simulink model "Sim_Helikopter_FB_VS"  (R2020b)
settings: Solver=ode113  StartTime=0.0  StopTime=50  RelTol=1e-2  EnableMultiTasking=on
PostLoadFcn:
  | , if any(exist('dsrtsu_mdlpostloadfcn', 'file') == [2, 3, 6]), try dsrtsu_mdlpostloadfcn('Execute', bdroot); catch fprintf('Error in PostLoadFcn (dsrtsu_mdlpostloadfcn) for model "%s":\n %s\n', bdroot, lasterr); end, end,
values from neighbouring files (symbols this model uses):
  Ta = 1e-3    (= 0.001)    [Initialisierung_bitte_vervollstaendigen.m]
undefined symbols (not defined in the file or in its folder): fbvsPar, initCond, sysPar
settings Model: DSRTSU_INTERNAL_RTI_VER=480  DSRTSU_INTERNAL_RTI_TYPE=rti1202  DSRTSU_INTERNAL_RTIFPGA=70  ExtModeArmWhenConnect=off  Creator=tk  LastModifiedBy=simon
settings DataIOCC: LimitDataPoints=on  SaveFormat=Array  SignalLoggingSaveFormat=ModelDataLogs  ReturnWorkspaceOutputs=off  SignalLoggingName=sigsOut
settings OptimizationCC: ConditionallyExecuteInputs=off  OptimizeBlockIOStorage=off  BufferReuse=off  GlobalBufferReuse=off  ExpressionFolding=off  ExpressionDepthLimit=2147483647  LocalBlockOutputs=off  InitFltsAndDblsToZero=on  LifeSpan=inf  OptimizeDataStoreBuffers=off  BusAssignmentInplaceUpdate=off
settings DebuggingCC: SaveWithParameterizedLinksMsg=none  UnderspecifiedInitializationDetection=Classic  MergeDetectMultiDrivingBlocksExec=none  SignalResolutionControl=TryResolveAllWithWarning  MultiTaskDSMMsg=warning  MultiTaskCondExecSysMsg=none  FcnCallInpInsideContextMsg=warning  AllowSymbolicDim=off  StateNameClashWarn=warning  SFUnexpectedBacktrackingDiag=warning  SFNoUnconditionalDefaultTransitionDiag=warning  SFExecutionAtInitializationDiag=none  ArithmeticOperatorsInVariantConditions=warning
settings HardwareCC: ProdBitPerPointer=32  ProdBitPerSizeT=32  ProdBitPerPtrDiffT=32  ProdLargestAtomicFloat=None  ProdIntDivRoundTo=Undefined  ProdEndianess=Unspecified  ProdWordSize=32  ProdHWDeviceType=32-bit Generic  TargetBitPerLong=64  TargetBitPerPointer=64  TargetBitPerSizeT=64  TargetBitPerPtrDiffT=64  TargetLongLongMode=on  TargetIntDivRoundTo=Zero  TargetEndianess=LittleEndian  TargetWordSize=64  TargetHWDeviceType=MATLAB Host  ProdEqTarget=off
settings ModelReferenceCC: PropagateSignalLabelsOutOfModel=off
settings SFSimCC: SimUseLocalCustomCode=off  SimParseCustomCode=off  CustomCodeUndefinedFunction=UseInterfaceOnly
settings RTWCC: Description=S-function Target  SystemTargetFile=rtwsfcn.tlc  TemplateMakefile=rtwsfcn_default_tmf  RetainRTWFile=on  RTWUseLocalCustomCode=off  RTWCompilerOptimization=on
settings CodeAppCC: StateflowObjectComments=on
settings STFCustomTargetCC: ModelReferenceCompliant=off  CompOptLevelCompliant=on  ConcurrentExecutionCompliant=off  MATLABClassNameForMDSCustomization=Simulink.SoftwareTarget.TargetSpecificTriggerConfigurationBase  CPPClassGenCompliant=off  SystemTargetFile=rtwsfcn.tlc
settings ConfigComp: CovMetricSettings=dw  CovSaveCumulativeToWorkspaceVar=on  CovSaveSingleToWorkspaceVar=on  CovExternalEMLEnable=off

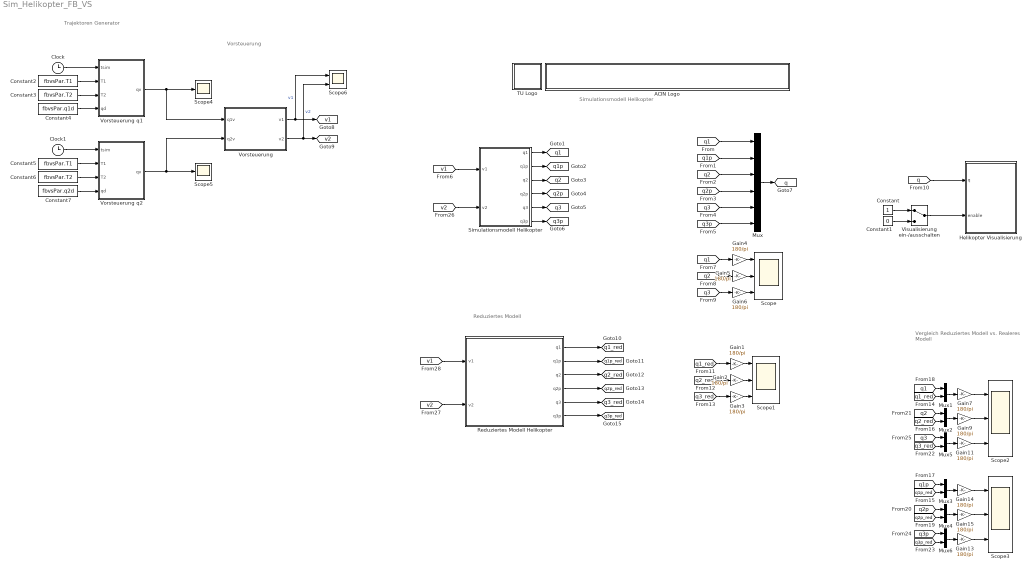
== system Sim_Helikopter_FB_VS ==
  note: Simulationsmodell Helikopter
  note: Reduziertes Modell
  note: Vergleich
      | Reduziertes Modell vs.
      | Realeres Modell
  note: Trajektoren
      | Generator
  note: Vorsteuerung
  ACIN Logo : Subsystem
      mask init:
      | s = get_param(gcb,'UserData');
      mask Display:
      | image(s.logo,[0 0 439 45]);
      | %axis image
  Clock : Clock
  Clock1 : Clock
  Constant : Constant
  Constant1 : Constant  Value=0
  Constant2 : Constant  Value=fbvsPar.T1
  Constant3 : Constant  Value=fbvsPar.T2
  Constant4 : Constant  Value=fbvsPar.q1d
  Constant5 : Constant  Value=fbvsPar.T1
  Constant6 : Constant  Value=fbvsPar.T2
  Constant7 : Constant  Value=fbvsPar.q2d
  Gain{1..7,9,11,13..15} (12 alike) : Gain  Gain=180/pi  SaturateOnIntegerOverflow=on  OutDataTypeStr=Inherit: Same as input  ParamDataTypeStr=Inherit: Same as input
  Helikopter Visualisierung : MATLAB Function  TreatAsAtomicUnit=on
  Mux : Mux  Inputs=6
  Mux{1..6} (6 alike) : Mux  Inputs=2
  Reduziertes Modell Helikopter : MATLAB Function  TreatAsAtomicUnit=on
  Scope{,1..3} (4 alike) : Scope  NumInputPorts=3
  Scope4 : Scope
  Scope5 : Scope
  Scope6 : Scope  NumInputPorts=2
  Simulationsmodell Helikopter : Subsystem
      settings: MinAlgLoopOccurrences=on
  TU Logo : Subsystem
      mask init:
      | s = get_param(gcb,'UserData');
      mask Display: image(s.logo,[0 0 45 45]);
  Visualisierung ein-/ausschalten : ManualSwitch
  Vorsteuerung : MATLAB Function  TreatAsAtomicUnit=on
  Vorsteuerung q1 : MATLAB Function  TreatAsAtomicUnit=on
  Vorsteuerung q2 : MATLAB Function  TreatAsAtomicUnit=on
  tag scope: q1=global, q1_red=global, q1p=global, q1p_red=global, q2=global, q2_red=global, q2p=global, q2p_red=global, q3=global, q3_red=global, q3p=global, q3p_red=global, q=global, v1=global, v2=global
  wires:
  Gain4/1 -> Scope/1
  Gain5/1 -> Scope/2
  Gain6/1 -> Scope/3
  Vorsteuerung/1(v1) -> Scope6/1, [v1]  "v1"
  Vorsteuerung/2(v2) -> Scope6/2, [v2]  "v2"
  Simulationsmodell Helikopter/1(q1) -> [q1]
  Simulationsmodell Helikopter/2(q1p) -> [q1p]
  Simulationsmodell Helikopter/3(q2) -> [q2]
  Simulationsmodell Helikopter/4(q2p) -> [q2p]
  Simulationsmodell Helikopter/5(q3) -> [q3]
  Simulationsmodell Helikopter/6(q3p) -> [q3p]
  Mux/1 -> [q]
  [q1] -> Mux/1
  [q1p] -> Mux/2
  [q2] -> Mux/3
  [q2p] -> Mux/4
  [q3] -> Mux/5
  [q3p] -> Mux/6
  [q1] -> Gain4/1
  [q2] -> Gain5/1
  [q3] -> Gain6/1
  Visualisierung ein-/ausschalten/1 -> Helikopter Visualisierung/2(enable)
  Constant/1 -> Visualisierung ein-/ausschalten/1
  [q] -> Helikopter Visualisierung/1(q)
  Constant1/1 -> Visualisierung ein-/ausschalten/2
  Reduziertes Modell Helikopter/1(q1) -> [q1_red]
  Reduziertes Modell Helikopter/2(q1p) -> [q1p_red]
  Reduziertes Modell Helikopter/3(q2) -> [q2_red]
  Reduziertes Modell Helikopter/4(q2p) -> [q2p_red]
  Reduziertes Modell Helikopter/5(q3) -> [q3_red]
  Reduziertes Modell Helikopter/6(q3p) -> [q3p_red]
  Gain1/1 -> Scope1/1
  [q1_red] -> Gain1/1
  Gain2/1 -> Scope1/2
  [q2_red] -> Gain2/1
  [q3_red] -> Gain3/1
  Gain3/1 -> Scope1/3
  Gain7/1 -> Scope2/1
  Mux1/1 -> Gain7/1
  [q1_red] -> Mux1/2
  [q1p_red] -> Mux3/2
  [q1p] -> Mux3/1
  [q1] -> Mux1/1
  [q2] -> Mux2/1
  [q2p] -> Mux4/1
  [q2_red] -> Mux2/2
  [q2p_red] -> Mux4/2
  [q3p_red] -> Mux6/2
  [q3p] -> Mux6/1
  [q3_red] -> Mux5/2
  [q3] -> Mux5/1
  Mux2/1 -> Gain9/1
  Mux5/1 -> Gain11/1
  Gain9/1 -> Scope2/2
  Gain11/1 -> Scope2/3
  Gain15/1 -> Scope3/2
  Gain14/1 -> Scope3/1
  Gain13/1 -> Scope3/3
  Mux3/1 -> Gain14/1
  Mux4/1 -> Gain15/1
  Mux6/1 -> Gain13/1
  [v1] -> Simulationsmodell Helikopter/1(v1)
  [v2] -> Simulationsmodell Helikopter/2(v2)
  [v1] -> Reduziertes Modell Helikopter/1(v1)
  [v2] -> Reduziertes Modell Helikopter/2(v2)
  Clock/1 -> Vorsteuerung q1/1(tsim)
  Constant2/1 -> Vorsteuerung q1/2(T1)
  Constant3/1 -> Vorsteuerung q1/3(T2)
  Constant4/1 -> Vorsteuerung q1/4(qd)
  Constant6/1 -> Vorsteuerung q2/3(T2)
  Clock1/1 -> Vorsteuerung q2/1(tsim)
  Constant5/1 -> Vorsteuerung q2/2(T1)
  Constant7/1 -> Vorsteuerung q2/4(qd)
  Vorsteuerung q1/1(qv) -> Vorsteuerung/1(q1v), Scope4/1
  Vorsteuerung q2/1(qv) -> Vorsteuerung/2(q2v), Scope5/1

== system Sim_Helikopter_FB_VS/ACIN Logo ==

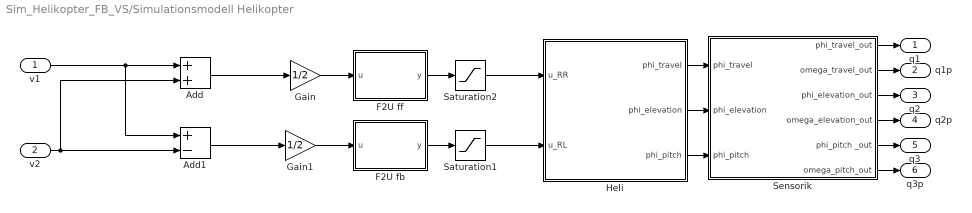
== system Sim_Helikopter_FB_VS/Simulationsmodell Helikopter ==
  v1 : Inport
  v2 : Inport  Port=2
  Add : Sum
  Add1 : Sum  Inputs=+-
  F2U fb : MATLAB Function  TreatAsAtomicUnit=on
  F2U ff : MATLAB Function  TreatAsAtomicUnit=on
  Gain : Gain  Gain=1/2
  Gain1 : Gain  Gain=1/2
  Heli : Subsystem
  Saturation1 : Saturate  UpperLimit=15  LowerLimit=-15
  Saturation2 : Saturate  UpperLimit=15  LowerLimit=-15
  Sensorik : Subsystem
  q1 : Outport  VectorParamsAs1DForOutWhenUnconnected=off
  q1p : Outport  Port=2  VectorParamsAs1DForOutWhenUnconnected=off
  q2 : Outport  Port=3  VectorParamsAs1DForOutWhenUnconnected=off
  q2p : Outport  Port=4  VectorParamsAs1DForOutWhenUnconnected=off
  q3 : Outport  Port=5  VectorParamsAs1DForOutWhenUnconnected=off
  q3p : Outport  Port=6  VectorParamsAs1DForOutWhenUnconnected=off
  wires:
  Saturation1/1 -> Heli/2(u_RL)
  Saturation2/1 -> Heli/1(u_RR)
  Heli/1(phi_travel) -> Sensorik/1(phi_travel)
  Heli/2(phi_elevation) -> Sensorik/2(phi_elevation)
  Heli/3(phi_pitch) -> Sensorik/3(phi_pitch)
  Sensorik/1(phi_travel_out) -> q1/1
  Sensorik/2(omega_travel_out) -> q1p/1
  Sensorik/3(phi_elevation_out) -> q2/1
  Sensorik/4(omega_elevation_out) -> q2p/1
  Sensorik/5(phi_pitch _out) -> q3/1
  Sensorik/6(omega_pitch_out) -> q3p/1
  v1/1 -> Add/1, Add1/1
  v2/1 -> Add/2, Add1/2
  Add/1 -> Gain/1
  Add1/1 -> Gain1/1
  Gain/1 -> F2U ff/1(u)
  Gain1/1 -> F2U fb/1(u)
  F2U ff/1(y) -> Saturation2/1
  F2U fb/1(y) -> Saturation1/1

== system Sim_Helikopter_FB_VS/TU Logo ==

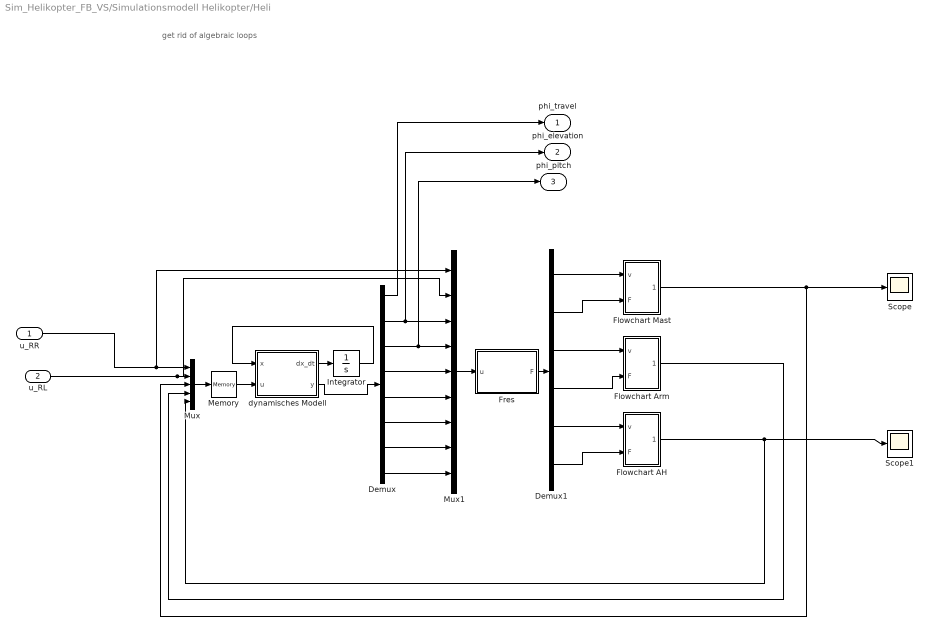
== system Sim_Helikopter_FB_VS/Simulationsmodell Helikopter/Heli ==
  note: get rid of algebraic loops
  u_RR : Inport
  u_RL : Inport  Port=2
  Demux : Demux  Outputs=8
      settings: DisplayOption=none
  Demux1 : Demux  Outputs=6
      settings: DisplayOption=none
  Flowchart AH : Subsystem
  Flowchart Arm : Subsystem
  Flowchart Mast : Subsystem
  Fres : MATLAB Function  TreatAsAtomicUnit=on
  Integrator : Integrator  InitialCondition=initCond
  Memory : Memory
  Mux : Mux  Inputs=5
  Mux1 : Mux  Inputs=9
  Scope : Scope
  Scope1 : Scope
  dynamisches Modell : MATLAB Function  TreatAsAtomicUnit=on
  phi_travel : Outport  VectorParamsAs1DForOutWhenUnconnected=off
  phi_elevation : Outport  Port=2  VectorParamsAs1DForOutWhenUnconnected=off
  phi_pitch : Outport  Port=3  VectorParamsAs1DForOutWhenUnconnected=off
  wires:
  Demux/1 -> phi_travel/1
  u_RR/1 -> Mux1/1, Mux/1
  u_RL/1 -> Mux1/2, Mux/2
  Demux1/6 -> Flowchart AH/2(F)
  Demux1/5 -> Flowchart AH/1(v)
  Demux1/4 -> Flowchart Arm/2(F)
  Demux1/3 -> Flowchart Arm/1(v)
  Demux1/2 -> Flowchart Mast/2(F)
  Demux1/1 -> Flowchart Mast/1(v)
  Fres/1(F) -> Demux1/1
  Mux1/1 -> Fres/1(u)
  Demux/2 -> Mux1/3, phi_elevation/1
  Demux/3 -> Mux1/4, phi_pitch/1
  Demux/4 -> Mux1/5
  Demux/5 -> Mux1/6
  Demux/6 -> Mux1/7
  Demux/7 -> Mux1/8
  Demux/8 -> Mux1/9
  dynamisches Modell/2(y) -> Demux/1
  Mux/1 -> Memory/1
  dynamisches Modell/1(dx_dt) -> Integrator/1
  Integrator/1 -> dynamisches Modell/1(x)
  Flowchart AH/1(Out1) -> Scope1/1, Mux/5
  Flowchart Arm/1(Out1) -> Mux/4
  Flowchart Mast/1(Out1) -> Mux/3, Scope/1
  Memory/1 -> dynamisches Modell/2(u)

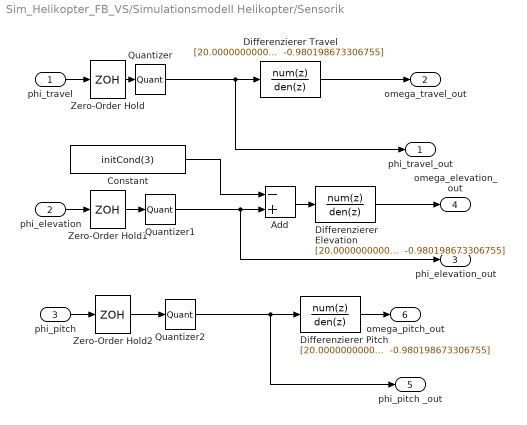
== system Sim_Helikopter_FB_VS/Simulationsmodell Helikopter/Sensorik ==
  phi_travel : Inport
  phi_elevation : Inport  Port=2
  phi_pitch : Inport  Port=3
  Add : Sum  Inputs=-+
  Constant : Constant  Value=initCond(3)
  Differenzierer Elevation : DiscreteTransferFcn  Numerator=[20.000000000000000 -19.999999999999996]  Denominator="[1.000000000000000  -0.980198673306755]"  SampleTime=1e-3
  Differenzierer Pitch : DiscreteTransferFcn  Numerator=[20.000000000000000 -19.999999999999996]  Denominator="[1.000000000000000  -0.980198673306755]"  SampleTime=1e-3
  Differenzierer Travel : DiscreteTransferFcn  Numerator=[20.000000000000000 -19.999999999999996]  Denominator="[1.000000000000000  -0.980198673306755]"  SampleTime=1e-3
  Quantizer : Quantizer  QuantizationInterval=2*pi/2^13
  Quantizer1 : Quantizer  QuantizationInterval=2*pi/4096
  Quantizer2 : Quantizer  QuantizationInterval=2*pi/4096
  Zero-Order Hold : ZeroOrderHold  SampleTime=1e-3
  Zero-Order Hold1 : ZeroOrderHold  SampleTime=1e-3
  Zero-Order Hold2 : ZeroOrderHold  SampleTime=1e-3
  phi_travel_out : Outport  VectorParamsAs1DForOutWhenUnconnected=off
  omega_travel_out : Outport  Port=2  VectorParamsAs1DForOutWhenUnconnected=off
  phi_elevation_out : Outport  Port=3  VectorParamsAs1DForOutWhenUnconnected=off
  omega_elevation_out : Outport  Port=4  VectorParamsAs1DForOutWhenUnconnected=off
  phi_pitch _out : Outport  Port=5  VectorParamsAs1DForOutWhenUnconnected=off
  omega_pitch_out : Outport  Port=6  VectorParamsAs1DForOutWhenUnconnected=off
  wires:
  Add/1 -> Differenzierer Elevation/1
  Constant/1 -> Add/1
  Zero-Order Hold/1 -> Quantizer/1
  Quantizer/1 -> Differenzierer Travel/1, phi_travel_out/1
  Zero-Order Hold1/1 -> Quantizer1/1
  Quantizer1/1 -> Add/2, phi_elevation_out/1
  Zero-Order Hold2/1 -> Quantizer2/1
  Quantizer2/1 -> phi_pitch _out/1, Differenzierer Pitch/1
  Differenzierer Travel/1 -> omega_travel_out/1
  phi_travel/1 -> Zero-Order Hold/1
  Differenzierer Elevation/1 -> omega_elevation_out/1
  phi_elevation/1 -> Zero-Order Hold1/1
  Differenzierer Pitch/1 -> omega_pitch_out/1
  phi_pitch/1 -> Zero-Order Hold2/1

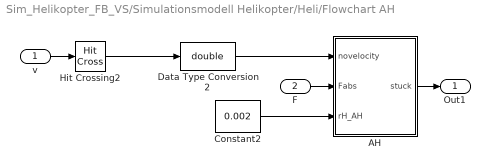
== system Sim_Helikopter_FB_VS/Simulationsmodell Helikopter/Heli/Flowchart AH ==
  v : Inport
  F : Inport  Port=2
  AH : Stateflow chart  TreatAsAtomicUnit=on
  Constant2 : Constant  Value=0.002
  Data Type Conversion2 : DataTypeConversion  OutDataTypeStr=double  SaturateOnIntegerOverflow=on  RndMeth=Zero
  Hit Crossing2 : HitCross  ZeroCross=off
  Out1 : Outport  VectorParamsAs1DForOutWhenUnconnected=off
  wires:
  AH/1(stuck) -> Out1/1
  F/1 -> AH/2(Fabs)
  v/1 -> Hit Crossing2/1
  Constant2/1 -> AH/3(rH_AH)
  Data Type Conversion2/1 -> AH/1(novelocity)
  Hit Crossing2/1 -> Data Type Conversion2/1

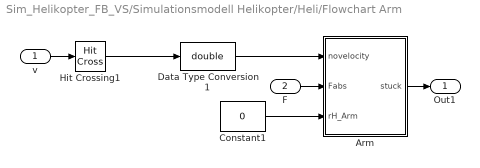
== system Sim_Helikopter_FB_VS/Simulationsmodell Helikopter/Heli/Flowchart Arm ==
  v : Inport
  F : Inport  Port=2
  Arm : Stateflow chart  TreatAsAtomicUnit=on
  Constant1 : Constant  Value=0
  Data Type Conversion1 : DataTypeConversion  OutDataTypeStr=double  SaturateOnIntegerOverflow=on  RndMeth=Zero
  Hit Crossing1 : HitCross  ZeroCross=off
  Out1 : Outport  VectorParamsAs1DForOutWhenUnconnected=off
  wires:
  Arm/1(stuck) -> Out1/1
  F/1 -> Arm/2(Fabs)
  v/1 -> Hit Crossing1/1
  Hit Crossing1/1 -> Data Type Conversion1/1
  Data Type Conversion1/1 -> Arm/1(novelocity)
  Constant1/1 -> Arm/3(rH_Arm)

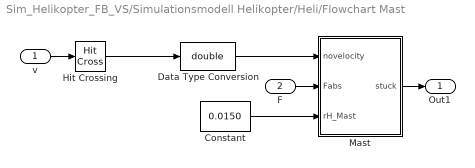
== system Sim_Helikopter_FB_VS/Simulationsmodell Helikopter/Heli/Flowchart Mast ==
  v : Inport
  F : Inport  Port=2
  Constant : Constant  Value=0.0150
  Data Type Conversion : DataTypeConversion  OutDataTypeStr=double  SaturateOnIntegerOverflow=on  RndMeth=Zero
  Hit Crossing : HitCross  ZeroCross=off
  Mast : Stateflow chart  TreatAsAtomicUnit=on
  Out1 : Outport  VectorParamsAs1DForOutWhenUnconnected=off
  wires:
  Mast/1(stuck) -> Out1/1
  F/1 -> Mast/2(Fabs)
  v/1 -> Hit Crossing/1
  Constant/1 -> Mast/3(rH_Mast)
  Data Type Conversion/1 -> Mast/1(novelocity)
  Hit Crossing/1 -> Data Type Conversion/1

== matlab function Sim_Helikopter_FB_VS/Simulationsmodell Helikopter/Heli/dynamisches Modell ==
  data: x input; u input; dx_dt output; p parameter; y output
function [dx_dt, y]= fcn(x, u, p)
%#codegen

[dx_dt, y] = heli_haft_mfun(x,u,p);

== matlab function Sim_Helikopter_FB_VS/Helikopter Visualisierung ==
  settings: updateMethod=DISCRETE  sampleTime=0.1
  data: q input; enable input
function visualization(q, enable)
  %Die Framerate wird durch die Sampling Time des Blocks vorgegeben.

  persistent ini; if isempty(ini);    ini = 0;    end
  persistent z12; if isempty(z12);    z12 = 1;    end
  persistent x23; if isempty(x23);    x23 = 1;    end
  persistent xh;  if isempty(xh);     xh = 1;     end
  persistent yh;  if isempty(yh);     yh = 1;     end
  persistent zh;  if isempty(zh);     zh = 1;     end
  persistent ph;  if isempty(ph);     ph = 1;     end
  
  if ~ini
    if(enable)
      h=figure(100);
      clf('reset');
      plot3(-2, -2, 0);
      plot3( 2,  2, 0);
      plot3(-2,  2, 0);
      plot3( 2, -2, 0);
      axis([-2 2 -2 2 0 1]);
      xlabel('x');
      ylabel('y');
      zlabel('-z');

      r  = 0.1;
      yn = 0.2:0.01:0.4;
      yp = 0.4:-0.01:0.2;
      a  = abs(r^2 - (yn - 0.3).^2);
      xn = -sqrt(a);
      xp =  sqrt(a);

      y2 = [yn'; yp'];
      x2 = [xn'; xp'];
      z2 = zeros(size(x2));

      yn = -0.2:-0.01:-0.4;
      yp = -0.4:0.01:-0.2;
      b  = abs(r^2 - (yn + 0.3).^2);
      xn = -sqrt(b);
      xp =  sqrt(b);

      y1 = [yn'; yp'];
      x1 = [xn'; xp'];
      z1 = zeros(size(x1));

      xh = [x1', x2'];
      yh = [y1', y2'];
      zh = [z1', z2'];
      ph = [xh; yh; zh; ones(size(zh))];
    else
      h=findobj('type','figure','Number',100);
      if(~isempty(h))
        close(h);
      end
    end
    ini = 1;
  end
  
  if(enable)
    q1=q(1);
    q2=q(3);
    q3=q(5);
    
    T02 = [-sin(q1) * cos(q2) -cos(q1) -sin(q1) * sin(q2) 0; cos(q1) * cos(q2) -sin(q1) cos(q1) * sin(q2) 0; -sin(q2) 0 cos(q2) z12; 0 0 0 1;];
    T03 = [-sin(q1) * cos(q2) cos(q1) * cos(q3) + sin(q1) * sin(q2) * sin(q3) -cos(q1) * sin(q3) + sin(q1) * sin(q2) * cos(q3) -sin(q1) * cos(q2) * x23; cos(q1) * cos(q2) sin(q1) * cos(q3) - cos(q1) * sin(q2) * sin(q3) -sin(q1) * sin(q3) - cos(q1) * sin(q2) * cos(q3) cos(q1) * cos(q2) * x23; -sin(q2) -cos(q2) * sin(q3) -cos(q2) * cos(q3) -sin(q2) * x23 + z12; 0 0 0 1;];

    clf('reset');
    % Nullzeiger
    xn = [0;1];
    yn = [0;0];
    zn = [0;0];
    plot3(xn, yn, zn);
    hold on;
    grid on;

    % Staender
    p0 = [0; 0; 0];
    p1 = [0; 0; 1];    
    lines = [p0';p1'];
    xs = lines(1:2,1);
    ys = lines(1:2,2);
    zs = lines(1:2,3);
    plot3(xs, ys, zs);

    % Balken
    p0 = T02*[1; 0; 0; 1];
    p1 = T02*[-1; 0; 0; 1];    
    lines = [p0(1:3)';p1(1:3)'];
    xb = lines(1:2,1);
    yb = lines(1:2,2);
    zb = lines(1:2,3);
    plot3(xb, yb, zb);

    % Helicopter
    lines = T03*ph;% [0; 0.2; 0; 1];
    % p1 = T03*[0; -0.2; 0; 1];    
    % lines = [p0(1:3)';p1(1:3)'];
    xh = lines(1,:);
    yh = lines(2,:);
    zh = lines(3,:);
    plot3(xh, yh, zh);

    plot3(-2, -2, 0);
    plot3( 2,  2, 0);
    plot3(-2,  2, 0);
    plot3( 2, -2, 0);
    axis([-2 2 -2 2 0 2]);

    drawnow
  end
end

== matlab function Sim_Helikopter_FB_VS/Vorsteuerung q2 ==
  data: tsim input; qv output; T1 input; T2 input; qd input
function qv = fcn(tsim,T1,T2,qd)

if(tsim <= T1)
    q10 = qd(1);
    q1T = qd(2);
    T = T1;
    t = tsim;
elseif(tsim <= T1+T2)
    q10 = qd(2);
    q1T = qd(3);
    T = T2;
    t = tsim-T1;
else
    q10 = 0;
    q1T = 0;
    T = 1;
    t = tsim-T1-T2;
end

if(tsim >= T1+T2)
    q1 = qd(3);
    q1p = 0;
    q1pp = 0;
    q1ppp = 0;
    q1pppp = 0;
else
    q1 = q10 + (q1T - q10) * (126 * t ^ 5 / T ^ 5 - 420 * t ^ 6 / T ^ 6 + 540 * t ^ 7 / T ^ 7 - 315 * t ^ 8 / T ^ 8 + 70 * t ^ 9 / T ^ 9);
    q1p = (q1T - q10) * (630 * t ^ 4 / T ^ 5 - 2520 * t ^ 5 / T ^ 6 + 3780 * t ^ 6 / T ^ 7 - 2520 * t ^ 7 / T ^ 8 + 630 * t ^ 8 / T ^ 9);
    q1pp = (q1T - q10) * (2520 * t ^ 3 / T ^ 5 - 12600 * t ^ 4 / T ^ 6 + 22680 * t ^ 5 / T ^ 7 - 17640 * t ^ 6 / T ^ 8 + 5040 * t ^ 7 / T ^ 9);
    q1ppp = (q1T - q10) * (7560 * t ^ 2 / T ^ 5 - 50400 * t ^ 3 / T ^ 6 + 113400 * t ^ 4 / T ^ 7 - 105840 * t ^ 5 / T ^ 8 + 35280 * t ^ 6 / T ^ 9);
    q1pppp = (q1T - q10) * (15120 * t / T ^ 5 - 151200 * t ^ 2 / T ^ 6 + 453600 * t ^ 3 / T ^ 7 - 529200 * t ^ 4 / T ^ 8 + 211680 * t ^ 5 / T ^ 9);
end

qv = [q1;q1p;q1pp;q1ppp;q1pppp];

== matlab function Sim_Helikopter_FB_VS/Simulationsmodell Helikopter/F2U ff ==
  data: u input; y output
function y = fcn(u)
%#codegen

y = F2U(u(1));

== stateflow chart Sim_Helikopter_FB_VS/Simulationsmodell Helikopter/Heli/Flowchart AH/AH ==
  state stuck/
    entry: stuck=1;
  state sliding/
    entry: stuck=0;
  (default) -> stuck
  sliding -> stuck : [novelocity & fabs(Fabs)<rH_AH]
  stuck -> sliding : [fabs(Fabs)>rH_AH]
  data: novelocity input boolean; Fabs input double; stuck output double; rH_AH input double

== stateflow chart Sim_Helikopter_FB_VS/Simulationsmodell Helikopter/Heli/Flowchart Arm/Arm ==
  state stuck/
    entry: stuck=1;
  state sliding/
    entry: stuck=0;
  (default) -> stuck
  sliding -> stuck : [novelocity & fabs(Fabs)<rH_Arm]
  stuck -> sliding : [fabs(Fabs)>rH_Arm]
  data: novelocity input boolean; Fabs input double; stuck output double; rH_Arm input double

== matlab function Sim_Helikopter_FB_VS/Vorsteuerung ==
  data: q1v input; v1 output; q2v input; v2 output; sysPar parameter
function [v1,v2] = FLATreg(q1v,q2v,sysPar)

% Systemparameter
a1 = sysPar.a1;
a2 = sysPar.a2;
a3 = sysPar.a3;
b1 = sysPar.b1;
b2 = sysPar.b2;
b3 = sysPar.b3;

% Sollwerte q1
q1 = q1v(1);
q1p = q1v(2);
q1pp = q1v(3);
q1ppp = q1v(4);
q1pppp = q1v(5);

% Sollwerte q2
q2 = q2v(1);
q2p = q2v(2);
q2pp = q2v(3);
q2ppp = q2v(4);
q2pppp = q2v(5);

% Steuergesetz
v1 = -0.1e1 / b2 * (a1 * sin(q2) + a2 * cos(q2) - q2pp) * sqrt(b2 ^ 2 * q1pp ^ 2 / b1 ^ 2 / cos(q2) ^ 2 / (a1 * sin(q2) + a2 * cos(q2) - q2pp) ^ 2 + 0.1e1);
v2 = -(-a3 * b2 * q1pp / b1 / (a1 * sin(q2) + a2 * cos(q2) - q2pp) * (b2 ^ 2 * q1pp ^ 2 / b1 ^ 2 / cos(q2) ^ 2 / (a1 * sin(q2) + a2 * cos(q2) - q2pp) ^ 2 + 0.1e1) ^ (-0.1e1 / 0.2e1) + (b2 * q1pppp / b1 / cos(q2) / (a1 * sin(q2) + a2 * cos(q2) - q2pp) + 0.2e1 * b2 * q1ppp / b1 / cos(q2) ^ 2 / (a1 * sin(q2) + a2 * cos(q2) - q2pp) * q2p * sin(q2) - 0.2e1 * b2 * q1ppp / b1 / cos(q2) / (a1 * sin(q2) + a2 * cos(q2) - q2pp) ^ 2 * (a1 * q2p * cos(q2) - a2 * q2p * sin(q2) - q2ppp) + 0.2e1 * b2 * q1pp / b1 / cos(q2) ^ 3 / (a1 * sin(q2) + a2 * cos(q2) - q2pp) * q2p ^ 2 * sin(q2) ^ 2 - 0.2e1 * b2 * q1pp / b1 / cos(q2) ^ 2 / (a1 * sin(q2) + a2 * cos(q2) - q2pp) ^ 2 * q2p * sin(q2) * (a1 * q2p * cos(q2) - a2 * q2p * sin(q2) - q2ppp) + b2 * q1pp / b1 / cos(q2) ^ 2 / (a1 * sin(q2) + a2 * cos(q2) - q2pp) * q2pp * sin(q2) + b2 * q1pp / b1 / cos(q2) / (a1 * sin(q2) + a2 * cos(q2) - q2pp) * q2p ^ 2 + 0.2e1 * b2 * q1pp / b1 / cos(q2) / (a1 * sin(q2) + a2 * cos(q2) - q2pp) ^ 3 * (a1 * q2p * cos(q2) - a2 * q2p * sin(q2) - q2ppp) ^ 2 - b2 * q1pp / b1 / cos(q2) / (a1 * sin(q2) + a2 * cos(q2) - q2pp) ^ 2 * (a1 * q2pp * cos(q2) - a1 * q2p ^ 2 * sin(q2) - a2 * q2pp * sin(q2) - a2 * q2p ^ 2 * cos(q2) - q2pppp)) / (b2 ^ 2 * q1pp ^ 2 / b1 ^ 2 / cos(q2) ^ 2 / (a1 * sin(q2) + a2 * cos(q2) - q2pp) ^ 2 + 0.1e1) - (b2 * q1ppp / b1 / cos(q2) / (a1 * sin(q2) + a2 * cos(q2) - q2pp) + b2 * q1pp / b1 / cos(q2) ^ 2 / (a1 * sin(q2) + a2 * cos(q2) - q2pp) * q2p * sin(q2) - b2 * q1pp / b1 / cos(q2) / (a1 * sin(q2) + a2 * cos(q2) - q2pp) ^ 2 * (a1 * q2p * cos(q2) - a2 * q2p * sin(q2) - q2ppp)) / (b2 ^ 2 * q1pp ^ 2 / b1 ^ 2 / cos(q2) ^ 2 / (a1 * sin(q2) + a2 * cos(q2) - q2pp) ^ 2 + 0.1e1) ^ 2 * (0.2e1 * b2 ^ 2 * q1pp / b1 ^ 2 / cos(q2) ^ 2 / (a1 * sin(q2) + a2 * cos(q2) - q2pp) ^ 2 * q1ppp + 0.2e1 * b2 ^ 2 * q1pp ^ 2 / b1 ^ 2 / cos(q2) ^ 3 / (a1 * sin(q2) + a2 * cos(q2) - q2pp) ^ 2 * q2p * sin(q2) - 0.2e1 * b2 ^ 2 * q1pp ^ 2 / b1 ^ 2 / cos(q2) ^ 2 / (a1 * sin(q2) + a2 * cos(q2) - q2pp) ^ 3 * (a1 * q2p * cos(q2) - a2 * q2p * sin(q2) - q2ppp))) / b3;

end

== stateflow chart Sim_Helikopter_FB_VS/Simulationsmodell Helikopter/Heli/Flowchart Mast/Mast ==
  state stuck/
    entry: stuck=1;
  state sliding/
    entry: stuck=0;
  sliding -> stuck : [novelocity & fabs(Fabs)<rH_Mast]
  stuck -> sliding : [fabs(Fabs)>rH_Mast]
  (default) -> sliding
  data: novelocity input boolean; Fabs input double; stuck output double; rH_Mast input double

== matlab function Sim_Helikopter_FB_VS/Reduziertes Modell Helikopter ==
  settings: updateMethod=DISCRETE  sampleTime=Ta
  data: v1 input; q1 output; v2 input; q1p output; q2 output; q2p output; q3 output; q3p output; sysPar parameter; Ta parameter
function [q1,q1p,q2,q2p,q3,q3p] = fcn(v1,v2,sysPar,Ta)

persistent x;
if isempty(x)
    x=sysPar.x0;
end

% Zustände
q1 = x(1);
q1p = x(2);
q2 = x(3);
q2p = x(4);
q3 = x(5);
q3p = x(6);

% Parameter
a1 = sysPar.a1;
a2 = sysPar.a2;
a3 = sysPar.a3;
b1 = sysPar.b1;
b2 = sysPar.b2;
b3 = sysPar.b3;

% System
xp = [q1p b1 * cos(q2) * sin(q3) * v1 q2p a1 * sin(q2) + a2 * cos(q2) + b2 * cos(q3) * v1 q3p a3 * cos(q2) * sin(q3) + b3 * v2];

% Integrator
x = x + xp'*Ta;

% Ausgabe
q1 = x(1);
q1p = x(2);
q2 = x(3);
q2p = x(4);
q3 = x(5);
q3p = x(6);

== matlab function Sim_Helikopter_FB_VS/Vorsteuerung q1 ==
  data: tsim input; qv output; T1 input; T2 input; qd input
function qv = fcn(tsim,T1,T2,qd)

if(tsim <= T1)
    q10 = qd(1);
    q1T = qd(2);
    T = T1;
    t = tsim;
elseif(tsim <= T1+T2)
    q10 = qd(2);
    q1T = qd(3);
    T = T2;
    t = tsim-T1;
else
    q10 = 0;
    q1T = 0;
    T = 1;
    t = tsim-T1-T2;
end

if(tsim >= T1+T2)
    q1 = qd(3);
    q1p = 0;
    q1pp = 0;
    q1ppp = 0;
    q1pppp = 0;
else
    q1 = q10 + (q1T - q10) * (126 * t ^ 5 / T ^ 5 - 420 * t ^ 6 / T ^ 6 + 540 * t ^ 7 / T ^ 7 - 315 * t ^ 8 / T ^ 8 + 70 * t ^ 9 / T ^ 9);
    q1p = (q1T - q10) * (630 * t ^ 4 / T ^ 5 - 2520 * t ^ 5 / T ^ 6 + 3780 * t ^ 6 / T ^ 7 - 2520 * t ^ 7 / T ^ 8 + 630 * t ^ 8 / T ^ 9);
    q1pp = (q1T - q10) * (2520 * t ^ 3 / T ^ 5 - 12600 * t ^ 4 / T ^ 6 + 22680 * t ^ 5 / T ^ 7 - 17640 * t ^ 6 / T ^ 8 + 5040 * t ^ 7 / T ^ 9);
    q1ppp = (q1T - q10) * (7560 * t ^ 2 / T ^ 5 - 50400 * t ^ 3 / T ^ 6 + 113400 * t ^ 4 / T ^ 7 - 105840 * t ^ 5 / T ^ 8 + 35280 * t ^ 6 / T ^ 9);
    q1pppp = (q1T - q10) * (15120 * t / T ^ 5 - 151200 * t ^ 2 / T ^ 6 + 453600 * t ^ 3 / T ^ 7 - 529200 * t ^ 4 / T ^ 8 + 211680 * t ^ 5 / T ^ 9);
end

qv = [q1;q1p;q1pp;q1ppp;q1pppp];

== matlab function Sim_Helikopter_FB_VS/Simulationsmodell Helikopter/F2U fb ==
  data: u input; y output
function y = fcn(u)
%#codegen

y = F2U(u(1));

== matlab function Sim_Helikopter_FB_VS/Simulationsmodell Helikopter/Heli/Fres ==
  data: u input; F output; parameters parameter
function F = fcn(u, parameters)
%#codegen

F = Fout(u(1),u(2),u(3),u(4),u(5),u(6),u(7),u(8),u(9),parameters);
